simulink model "untitled"  (R2018b)
settings: Solver=VariableStepAuto  StartTime=0.0  StopTime=20  RelTol=1e-3
settings Model: Creator=Никита Волк  LastModifiedBy=Никита Волк

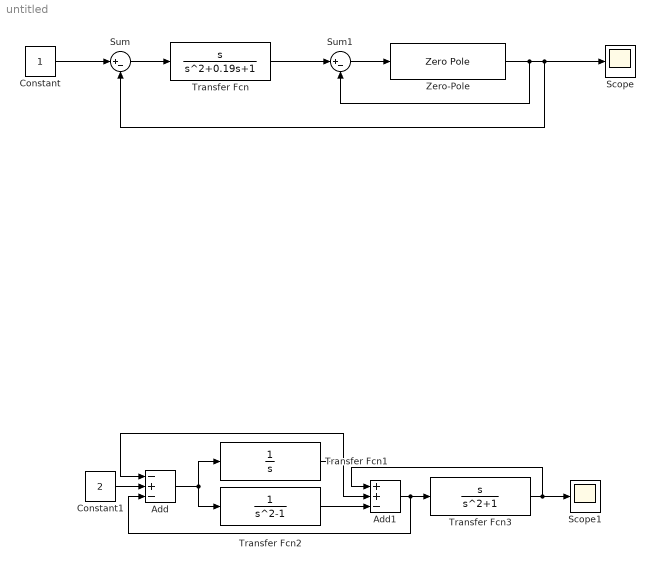
== system untitled ==
  Add : Sum  Inputs=-+-
  Add1 : Sum  Inputs=++-
  Constant : Constant
  Constant1 : Constant  Value=2
  Scope : Scope
  Scope1 : Scope
  Sum : Sum  Inputs=|+-
  Sum1 : Sum  Inputs=|+-
  Transfer Fcn : TransferFcn  Numerator=[1 0]  Denominator=[1 0.19 1]
  Transfer Fcn1 : TransferFcn  Denominator=[1 0]
  Transfer Fcn2 : TransferFcn  Denominator=[1 0 -1]
  Transfer Fcn3 : TransferFcn  Numerator=[1 0]  Denominator=[1 0 1]
  Zero-Pole : ZeroPole  Zeros=[0]  Poles=[-0.07 -1]
  wires:
  Sum1/1 -> Zero-Pole/1
  Zero-Pole/1 -> Scope/1, Sum/2, Sum1/2
  Transfer Fcn/1 -> Sum1/1
  Sum/1 -> Transfer Fcn/1
  Constant/1 -> Sum/1
  Constant1/1 -> Add/2
  Add/1 -> Transfer Fcn2/1, Transfer Fcn1/1
  Transfer Fcn1/1 -> Add/1, Add1/2
  Transfer Fcn2/1 -> Add1/3
  Transfer Fcn3/1 -> Scope1/1, Add1/1
  Add1/1 -> Transfer Fcn3/1, Add/3
